simulink model "MFWF_plant"  (R2025b)
settings: Solver=FixedStepAuto  StartTime=0  StopTime=100  FixedStep=0.001  MaxStep=0.1  RelTol=1e-3  EnableMultiTasking=on
settings Model: DataDictionary=topLevel.sldd  ModifiedByFormat=The MathWorks Inc.  Creator=The MathWorks, Inc.  LastModifiedBy=The MathWorks Inc.
settings SolverCC: AlgebraicLoopSolver=TrustRegion  AutoInsertRateTranBlk=on
settings DataIOCC: ReturnWorkspaceOutputs=off
settings OptimizationCC: BlockReduction=off  DefaultParameterBehavior=Inlined  BufferReuse=off  ExpressionDepthLimit=2147483647.0  LifeSpan=1
settings DebuggingCC: AlgebraicLoopMsg=none  UnderspecifiedInitializationDetection=Classic  MergeDetectMultiDrivingBlocksExec=none  FcnCallInpInsideContextMsg=warning  AllowSymbolicDim=off  StateNameClashWarn=warning  SFUnexpectedBacktrackingDiag=warning  SFNoUnconditionalDefaultTransitionDiag=warning  SFExecutionAtInitializationDiag=none  ArithmeticOperatorsInVariantConditions=warning
settings HardwareCC: ProdBitPerPointer=32.0  ProdBitPerSizeT=32.0  ProdBitPerPtrDiffT=32.0  ProdLargestAtomicFloat=None  ProdIntDivRoundTo=Undefined  ProdEndianess=Unspecified  ProdWordSize=32.0  ProdHWDeviceType=32-bit Generic
settings ModelReferenceCC: EnableRefExpFcnMdlSchedulingChecks=on  PropagateSignalLabelsOutOfModel=off
settings SFSimCC: SimUseLocalCustomCode=off  CustomCodeUndefinedFunction=UseInterfaceOnly
settings RTWCC: RTWUseLocalCustomCode=off  GPUComputeCapability=3.5  DLArmComputeVersion=19.05
settings CodeAppCC: StateflowObjectComments=on
settings GRTTargetCC: TargetLangStandard=C89/C90 (ANSI)  CombineOutputUpdateFcns=off  GRTInterface=on
settings ConfigComp: CovMetricSettings=dw  CovSaveCumulativeToWorkspaceVar=on  CovSaveSingleToWorkspaceVar=on  CovExternalEMLEnable=off  CovSFcnEnable=off
settings SimscapeCC: SimscapeLogDecimation=1  SimscapeLogDataHistory=5000

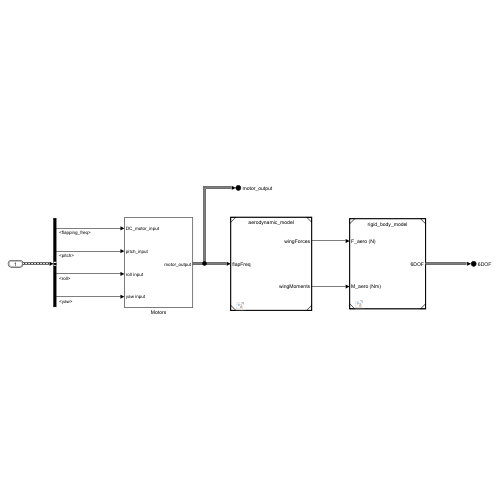
[thumbnail: Simulink's stored preview of the top-level diagram]
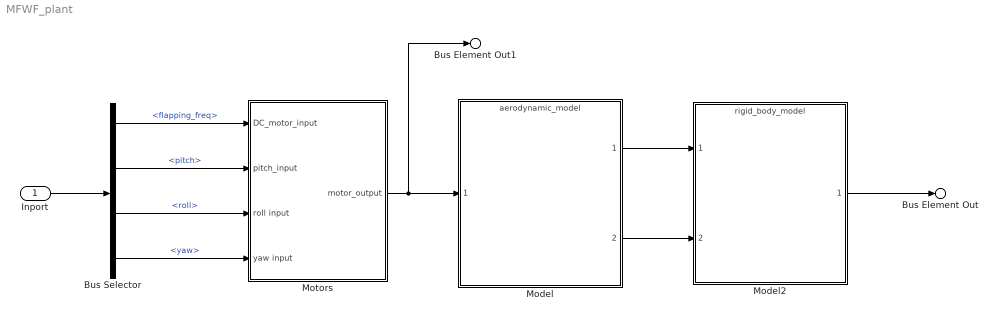
== system MFWF_plant ==
  Inport : Inport  OutDataTypeStr=Bus: motor_input  BusOutputAsStruct=on
  Bus Selector : BusSelector  OutputSignals=flapping_freq,pitch,roll,yaw
  Model : ModelReference  ModelNameDialog=aerodynamic_model  ParameterArgumentNames=cycleAvg  UsingDefaultArgumentValue=0  SimulationMode=Normal  ModelReferenceVersion=17.109
  Model2 : ModelReference  ModelNameDialog=rigid_body_model  SimulationMode=Normal  ModelReferenceVersion=17.57
  Motors : Subsystem  Description=Simulation of main DC motor and controlling servo motor actuators to approximate response from controller commands.
  Bus Element Out1 : Outport  PortName=motor_output
  Bus Element Out : Outport  Port=2  PortName=6DOF
  wires:
  Bus Selector/4 -> Motors/4(yaw input)  "<yaw>"
  Model2/1 -> Bus Element Out/1
  Motors/1(motor_output) -> Bus Element Out1/1, Model/1
  Model/1 -> Model2/1
  Model/2 -> Model2/2
  Inport/1 -> Bus Selector/1
  Bus Selector/3 -> Motors/3(roll input)  "<roll>"
  Bus Selector/1 -> Motors/1(DC_motor_input)  "<flapping_freq>"
  Bus Selector/2 -> Motors/2(pitch_input)  "<pitch>"

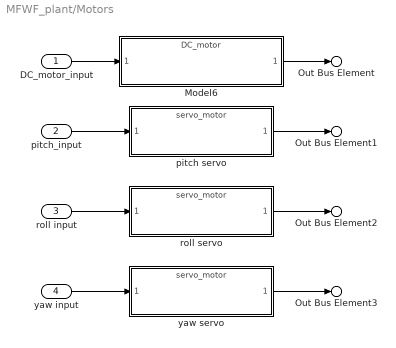
== system MFWF_plant/Motors ==
  DC_motor_input : Inport
  pitch_input : Inport  Port=2
  roll input : Inport  Port=3
  yaw input : Inport  Port=4
  Model6 : ModelReference  ModelNameDialog=DC_motor  SimulationMode=Normal  ModelReferenceVersion=8.25
  pitch servo : ModelReference  ModelNameDialog=servo_motor  SimulationMode=Normal  ModelReferenceVersion=17.2
  roll servo : ModelReference  ModelNameDialog=servo_motor  SimulationMode=Normal  ModelReferenceVersion=17.2
  yaw servo : ModelReference  ModelNameDialog=servo_motor  SimulationMode=Normal  ModelReferenceVersion=17.2
  Out Bus Element : Outport  PortName=motor_output  Element=flapping_freq
  Out Bus Element1 : Outport  PortName=motor_output  Element=pitch
  Out Bus Element2 : Outport  PortName=motor_output  Element=roll
  Out Bus Element3 : Outport  PortName=motor_output  Element=yaw
  wires:
  roll servo/1 -> Out Bus Element2/1
  pitch servo/1 -> Out Bus Element1/1
  yaw servo/1 -> Out Bus Element3/1
  pitch_input/1 -> pitch servo/1
  roll input/1 -> roll servo/1
  yaw input/1 -> yaw servo/1
  DC_motor_input/1 -> Model6/1
  Model6/1 -> Out Bus Element/1
